simulink model "A320_23b"  (R2024b)
settings: Solver=ode4  StartTime=0.0  StopTime=150  FixedStep=0.001  RelTol=1e-3
InitFcn:
  | % 清空工作区
  | % clear;
  | 
  | % 加载气动数据
  | load('engine_ct_table.mat'); % 或者是你那个存有气动数据的文件名
values from neighbouring files (symbols this model uses):
  a0 = 340.294    [basedata.m]
  alpha_CL_table = [ -3.150;  0.000;  0.139;  0.200;  0.260;  0.290;  0.320;  0.500;  3.150 ]    [basedata.m]
  alpha_Cm_table = [ -3.150; -0.800; -0.400; -0.200; -0.100;  0.000;  0.200;  0.230;  0.260;  0.290;  0.310;  0.400;  0.800;  3.150 ]    [basedata.m]
  alpha_Kde_table = [ -3.141593; -0.698132; -0.349066; -0.174533; -0.087266;  0.000000;  0.087266;  0.174533;  0.349066;  0.698132;  3.141593 ]    [basedata.m]
  b_ref = 35.799979    [basedata.m]
  c_gear = 2 .* damping_ratio .* sqrt(k_gear .* m_eff_gear)    [gear.m]
  c_ref = S_ref / b_ref    (= 3.41891172618)    [basedata.m]
  c_roll = [0.020, 0.018, 0.018]    [gear.m]
  CD0 = 0.01865    [basedata.m]
  CL_D0 = CL_D0_clean    (= 0.175)    [basedata.m]
  CL_table = [  0.000;  0.138;  1.320;  1.480;  1.760;  1.750;  1.600;  1.500;  0.000 ]    [basedata.m]
  Clb = 0.554    [basedata.m]
  Clda = -0.291    [basedata.m]
  CLde = -1.652    [basedata.m]
  Cldr = 0.476    [basedata.m]
  Clp = -2.078    [basedata.m]
  CLq = -57.116    [basedata.m]
  Clr = -2.621    [basedata.m]
  Cm_table = [  0.000; -2.402; -1.861; -0.842; -0.442;  0.000;  1.173;  1.337;  1.489;  1.723;  1.919;  2.276;  2.992;  0.000 ]    [basedata.m]
  Cmde = -11.78    [basedata.m]
  Cmq = -1245.917    [basedata.m]
  Cnb = 1.296    [basedata.m]
  Cnda = -0.007    [basedata.m]
  Cndr = 1.321    [basedata.m]
  Cnp = 0.742    [basedata.m]
  Cnr = -67.303    [basedata.m]
  CSb = -3.252    [basedata.m]
  CSdr = -2.793    [basedata.m]
  CSr = 17.395    [basedata.m]
  CT_ref = 1.3621132    [basedata.m]    (also in generate_engine_ct_table.m)
  CT_table = [      0.000000, 0.000000, 0.000000, 0.000000, 0.000000, 0.000000, 0.000000, 0.000000, 0.000000, 0.000000;      0.091741, 0.057020, 0.052029, 0.028096, -0.017284, -0.037284, -0.057077, -0.205841, -0.315399, -0.488717;      0.142810, 0.072215, 0.053026, 0.030404, -0.009593, -0.026571, -0.041999, -0.151328, -0.266204, -0.439028;      0.189837, 0.082322, 0.055050, 0.032748,  0.017389,  0.003990, -0.0 ...(+1815 chars)    [generate_engine_ct_table.m]
  CYp = 1.833    [basedata.m]
  da_max = 0.436332    [basedata.m]
  da_min = -da_max    (= -0.436332)    [basedata.m]
  de_max = 0.436332    [basedata.m]
  de_min = -0.296706    [basedata.m]
  Delta_CD_flap_tot = 0.1316    [basedata.m]
  Delta_CD_gear = 0.0372    [basedata.m]    (also in gear.m)
  Delta_CD_sp = 0.05775    [basedata.m]
  Delta_CL_flap_tot = 1.867    [basedata.m]
  Delta_CL_sp = -0.466875    [basedata.m]
  Delta_Cm_flap_tot = -0.084    [basedata.m]
  Delta_Cm_gear = 0.0022    [basedata.m]    (also in gear.m)
  Delta_Cm_sp = 0.023    [basedata.m]
  delta_flap_TE_max = 0.698132    [basedata.m]
  delta_flap_TE_tab = [ 0.000000;  0.087266;  0.174533;  0.261799;  0.349066;  0.698132 ]    [basedata.m]
  delta_gear_max = [0.573024, 0.523235, 0.523235]    [gear.m]
  delta_slat_LE_max = 0.471239    [basedata.m]
  delta_slat_LE_tab = [ 0.000000;  0.314159;  0.314334;  0.383972;  0.384147;  0.471239 ]    [basedata.m]
  DH = pi / 180    (= 0.0174532925199)    [basedata.m]
  dr_max = 0.436332    [basedata.m]
  dr_min = -dr_max    (= -0.436332)    [basedata.m]
  g = 9.80665    [basedata.m]
  ground_z = 0.0    (= 0)    [gear.m]
  H_B = H_R - R * cos(a1)    [landing_trajectory.m]
  H_C = H_R - R * cos(a2)    [landing_trajectory.m]
  H_climb_complete = 1000.0    (= 1000)    [landing.m]
  H_entry = 1001    [landing_trajectory.m]
  H_exp = 20    [landing_trajectory.m]
  HD = 180 / pi    (= 57.2957795131)    [basedata.m]
  I = [ Ixx, -Ixy, -Ixz ... (first row only)    [basedata.m]
  K_GE = 1.0    (= 1)    [basedata.m]
  K_gear = F_static_gear ./ (delta_static .^ spring_exp)    [gear.m]
  k_i_eff = 0.07447685    [basedata.m]
  Kde_table = [ -1.000;     0.050;     0.455;     0.853;     1.007;     1.000;     0.839;     0.693;     0.381;    -0.080;   -1.000 ]    [basedata.m]
  lamdaD_flap_TE_tab = [ 0.000;     0.300;     0.630;     0.850;     0.970;     0.939 ]    [basedata.m]
  lamdaD_slat_LE_tab = [ 1.000;     0.330;     0.630;     0.850;     0.970;     0.939 ]    [basedata.m]
  lamdaL_flap_TE_tab = [ 0.000;     0.010;     1.300;     1.300;     1.170;     1.000 ]    [basedata.m]
  lamdaL_slat_LE_tab = [ 1.000;     1.000;     1.000;     1.000;     1.000;     1.000 ]    [basedata.m]
  m = 42500.244    [basedata.m]
  Mach = [0, 0.1, 0.2, 0.3, 0.4, 0.5, 0.6, 0.7, 0.8, 0.9]    [generate_engine_ct_table.m]
  mu_brake = [0.0, 0.55, 0.55]    [gear.m]
  mu_lat = mu_gear    [gear.m]
  N1 = [        0,  20,  25,  30,  35,  40,  45,  50,  55,  60,       65,  70,  75,  80,  85,  90,  95, 100, 105, 110]    [generate_engine_ct_table.m]
  N1_idle = 19.6    [basedata.m]    (also in generate_engine_ct_table.m)
  N1_lim = 101.0    (= 101)    [basedata.m]    (also in generate_engine_ct_table.m)
  phi0 = 0.0    (= 0)    [landing.m]
  psi0 = 0.0    (= 0)    [landing.m]
  r_left_b = r_gear_b(:,2)    [gear.m]
  r_nose_b = r_gear_b(:,1)    [gear.m]
  r_right_b = r_gear_b(:,3)    [gear.m]
  rho0 = 1.225    [basedata.m]
  S_ref = 122.396968    [basedata.m]
  spoiler_max_air = 0.698132    [basedata.m]
  spring_exp = [2.05, 1.05, 1.05]    [gear.m]
  T_static = 120635.770206    [basedata.m]    (also in generate_engine_ct_table.m)
  theta0 = alpha_trim    [landing.m]
  V_app = 1.4 * Vs    [landing_trajectory.m]
  V_cruise = 234.072222    [basedata.m]
  v_eps = 0.20    (= 0.2)    [gear.m]
  V_flare = 1.4 * V_stall_full    (= 82.8255554)    [basedata.m]    (also in landing.m = 1.4 * V_stall_full)
  V_lat_ref = 0.20    (= 0.2)    [gear.m]
  V_min = 3    [landing.m]
  V_shallow = 1.2 * Vs    [landing_trajectory.m]
  wheel_radius = [0.381000, 0.584210, 0.584210]    [gear.m]
  WOW_on = 0.005    [gear.m]
  X_landing_start = -11500    [landing.m]
  Xg0 = -11500.0    (= -11500)    [landing.m]
  Yg0 = 100.0    (= 100)    [landing.m]
  Zg0 = -10000    [gear.m]    (also in landing.m = -1000)
undefined symbols (not defined in the file or in its folder): I_xz, I_yz, Ix_Iy, Iy_Iz, Iz_Ix
libraries: simulink x51, matrix_library x19
(part 1 of 3)
settings Model: SimulationMode=accelerator  Creator=34355  LastModifiedBy=34355

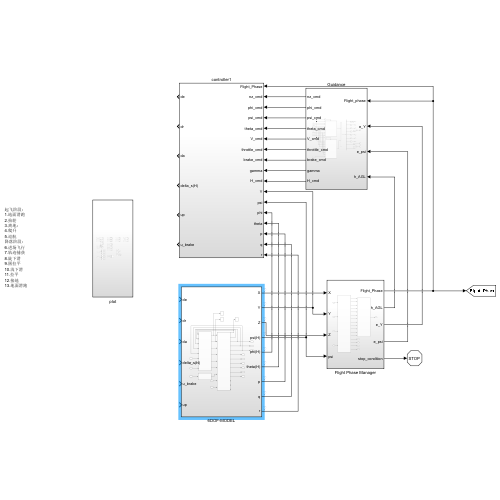
[thumbnail: Simulink's stored preview of the top-level diagram]
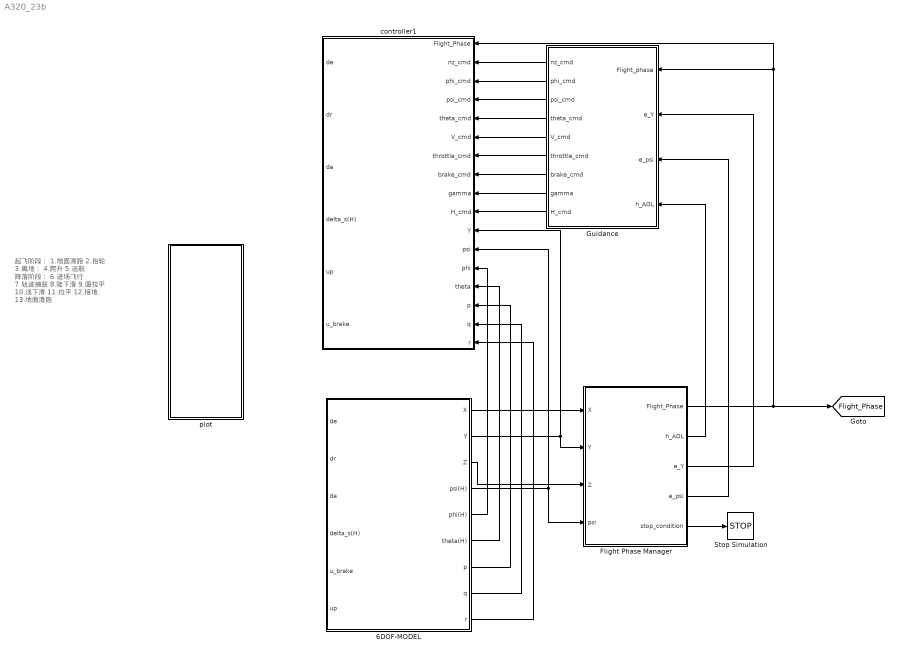
== system A320_23b ==
  note: 起飞阶段：
      | 1.地面滑跑
      | 2.抬轮
      | 3.离地：
      | 4.爬升
      | 5.巡航
      | 降落阶段：
      | 6.进场飞行
      | 7.轨迹捕获
      | 8.陡下滑
      | 9.圆拉平
      | 10.浅下滑
      | 11.拉平
      | 12.接地
      | 13.地面滑跑
  6DOF-MODEL : Subsystem
  Flight Phase Manager : Subsystem
  Guidance : Subsystem
  Stop Simulation : Stop
  controller1 : Subsystem
  plot : Subsystem
  tag scope: Flight_Phase=global
  wires:
  Flight Phase Manager/1(Flight_Phase) -> [Flight_Phase], Guidance/1(Flight_phase), controller1/1(Flight_Phase)
  Flight Phase Manager/3(e_Y) -> Guidance/2(e_Y)
  Flight Phase Manager/4(e_psi) -> Guidance/3(e_psi)
  Flight Phase Manager/2(h_AGL) -> Guidance/4(h_AGL)
  Guidance/1(nz_cmd) -> controller1/2(nz_cmd)
  Guidance/2(phi_cmd) -> controller1/3(phi_cmd)
  Guidance/4(theta_cmd) -> controller1/5(theta_cmd)
  Guidance/5(V_cmd) -> controller1/6(V_cmd)
  Guidance/6(throttle_cmd) -> controller1/7(throttle_cmd)
  Guidance/7(brake_cmd) -> controller1/8(brake_cmd)
  Guidance/8(gamma) -> controller1/9(gamma)
  Guidance/9(H_cmd) -> controller1/10(H_cmd)
  Flight Phase Manager/5(stop_condition) -> Stop Simulation/1
  Guidance/3(psi_cmd) -> controller1/4(psi_cmd)
  6DOF-MODEL/1(X) -> Flight Phase Manager/1(X)
  6DOF-MODEL/2(Y) -> controller1/11(Y), Flight Phase Manager/2(Y)
  6DOF-MODEL/3(Z) -> Flight Phase Manager/3(Z)
  6DOF-MODEL/4(psi(H)) -> Flight Phase Manager/4(psi), controller1/12(psi)
  6DOF-MODEL/5(phi(H)) -> controller1/13(phi)
  6DOF-MODEL/6(theta(H)) -> controller1/14(theta)
  6DOF-MODEL/7(p) -> controller1/15(p)
  6DOF-MODEL/8(q) -> controller1/16(q)
  6DOF-MODEL/9(r) -> controller1/17(r)

== system A320_23b/6DOF-MODEL ==
  de : Inport
  dr : Inport  Port=2
  da : Inport  Port=3
  delta_s(H) : Inport  Port=4
  u_brake : Inport  Port=5
  up : Inport  Port=6
  AERO-PARAMETER : Subsystem
  Scope : Scope
  Scope5 : Scope
  Scope6 : Scope
  动力学 : Subsystem
  发动机 : Subsystem
  X : Outport
  Y : Outport  Port=2
  Z : Outport  Port=3
  psi(H) : Outport  Port=4
  phi(H) : Outport  Port=5
  theta(H) : Outport  Port=6
  p : Outport  Port=7
  q : Outport  Port=8
  r : Outport  Port=9
  wires:
  动力学/1(alpha(D)) -> Scope/1, AERO-PARAMETER/1(alpha(D))
  发动机/1(T) -> 动力学/7(thrust)
  u_brake/1 -> 动力学/9(u_brake)
  AERO-PARAMETER/1(D) -> Scope6/1, 动力学/1(D)
  AERO-PARAMETER/2(L) -> Scope5/1, 动力学/2(L)
  AERO-PARAMETER/3(S) -> 动力学/3(S)
  AERO-PARAMETER/4(MX) -> 动力学/4(MX)
  AERO-PARAMETER/5(MY) -> 动力学/5(MY)
  AERO-PARAMETER/6(MZ) -> 动力学/6(MZ)
  delta_s(H)/1 -> 动力学/8(delta_s(H))
  动力学/2(beta(D)) -> AERO-PARAMETER/2(beta(D))
  动力学/3(p) -> p/1, AERO-PARAMETER/3(p(H))
  动力学/4(q) -> q/1, AERO-PARAMETER/4(q(H))
  动力学/5(r) -> r/1, AERO-PARAMETER/5(r(H))
  de/1 -> AERO-PARAMETER/6(de(D))
  dr/1 -> AERO-PARAMETER/7(dr(D))
  da/1 -> AERO-PARAMETER/8(da)
  动力学/7(Y) -> Y/1
  动力学/8(Z) -> Z/1
  动力学/11(psi(H)) -> psi(H)/1
  动力学/10(theta(H)) -> theta(H)/1
  动力学/6(X) -> X/1
  动力学/9(phi(H)) -> phi(H)/1
  up/1 -> 发动机/1(up)

== system A320_23b/Flight Phase Manager ==
  X : Inport
  Y : Inport  Port=2
  Z : Inport  Port=3
  psi : Inport  Port=4
  Data Pre-processing : Subsystem
  Phase Logic : Stateflow chart  TreatAsAtomicUnit=on
  Flight_Phase : Outport
  h_AGL : Outport  Port=2
  e_Y : Outport  Port=3
  e_psi : Outport  Port=4
  stop_condition : Outport  Port=5
  wires:
  X/1 -> Data Pre-processing/1(X)
  Y/1 -> Data Pre-processing/2(Y)
  Z/1 -> Data Pre-processing/3(Z)
  psi/1 -> Data Pre-processing/4(psi)
  Phase Logic/1(Flight_Phase) -> Flight_Phase/1
  Data Pre-processing/1(reach_VR) -> Phase Logic/1(reach_VR)
  Data Pre-processing/2(airborne) -> Phase Logic/2(airborne)
  Data Pre-processing/3(safe_climb) -> Phase Logic/3(safe_climb)
  Data Pre-processing/4(in_cruise) -> Phase Logic/4(in_cruise)
  Data Pre-processing/5(task_mode) -> Phase Logic/5(Task_Mode)
  Data Pre-processing/6(Trajectory_capture) -> Phase Logic/6(Trajectory_capture)
  Data Pre-processing/7(in_steep) -> Phase Logic/7(in_steep)
  Data Pre-processing/8(In_round) -> Phase Logic/8(in_round)
  Data Pre-processing/9(Slight decline) -> Phase Logic/9(Slight_decline)
  Data Pre-processing/10(in_flare) -> Phase Logic/10(in_Flare)
  Data Pre-processing/11(touch_ground) -> Phase Logic/11(touch_ground)
  Data Pre-processing/12(in_ground) -> Phase Logic/12(in_ground)
  Data Pre-processing/13(h_ALG) -> h_AGL/1
  Data Pre-processing/15(e_Y) -> e_Y/1
  Data Pre-processing/14(e_psi) -> e_psi/1
  Data Pre-processing/16(stop_condition) -> stop_condition/1

== system A320_23b/Guidance ==
  Flight_phase : Inport
  e_Y : Inport  Port=2
  e_psi : Inport  Port=3
  h_AGL : Inport  Port=4
  Bus Selector : BusSelector  OutputSignals=nz_cmd,phi_cmd,psi_cmd,theta_cmd,V_cmd,throttle_cmd,brake_cmd,H_cmd,gamma
  Compare To Constant : simulink/Logic and Bit Operations/Compare To Constant  relop=<=  const=5  OutDataTypeStr=boolean
  Compare To Constant1 : simulink/Logic and Bit Operations/Compare To Constant  relop=>  const=5  OutDataTypeStr=boolean
  Gain : Gain  Gain=HD
  Gain1 : Gain  Gain=HD
  Merge : Merge
  Rate Limiter : RateLimiter  RisingSlewLimit=1*DH  FallingSlewLimit=-1*DH  SampleTimeMode=inherited
  Rate Limiter1 : RateLimiter  RisingSlewLimit=10*DH  FallingSlewLimit=-10*DH  SampleTimeMode=inherited
  Rate Limiter2 : RateLimiter  RisingSlewLimit=10*DH  FallingSlewLimit=-10*DH  SampleTimeMode=inherited
  Rate Limiter3 : RateLimiter  RisingSlewLimit=0.8  FallingSlewLimit=-0.8  SampleTimeMode=inherited
  Saturation : Saturate  UpperLimit=2  LowerLimit=-2
  Saturation2 : Saturate  UpperLimit=1  LowerLimit=0
  Saturation3 : Saturate  UpperLimit=1  LowerLimit=0
  Saturation4 : Saturate  UpperLimit=250  LowerLimit=0
  Scope : Scope
  Scope8 : Scope
  Scope9 : Scope
  起飞阶段 : Subsystem
  降落阶段 : Subsystem
  nz_cmd : Outport
  phi_cmd : Outport  Port=2
  psi_cmd : Outport  Port=3
  theta_cmd : Outport  Port=4
  V_cmd : Outport  Port=5
  throttle_cmd : Outport  Port=6
  brake_cmd : Outport  Port=7
  gamma : Outport  Port=8
  H_cmd : Outport  Port=9
  wires:
  Bus Selector/5 -> Saturation4/1  "<V_cmd>"
  Bus Selector/4 -> Rate Limiter/1  "<theta_cmd>"
  Saturation4/1 -> V_cmd/1
  Bus Selector/7 -> Saturation3/1  "<brake_cmd>"
  Rate Limiter2/1 -> psi_cmd/1
  Saturation/1 -> Rate Limiter3/1
  Saturation3/1 -> brake_cmd/1
  Saturation2/1 -> throttle_cmd/1
  Merge/1 -> Bus Selector/1
  [vzg] -> 起飞阶段/8(vzg), 降落阶段/6(vzg)
  Rate Limiter/1 -> theta_cmd/1, Gain1/1
  Bus Selector/2 -> Rate Limiter1/1  "<phi_cmd>"
  Bus Selector/8 -> H_cmd/1, Scope9/1  "<H_cmd>"
  [theta_eular] -> 降落阶段/8(theta_eular), 起飞阶段/10(theta_eular)
  降落阶段/1(Cmd_Bus) -> Merge/2
  Bus Selector/1 -> Saturation/1  "<nz_cmd>"
  h_AGL/1 -> 起飞阶段/7(h_ALG), 降落阶段/2(h_AGL)
  [vxg] -> 降落阶段/9(Vg)
  [phi_eular] -> 起飞阶段/9(phi_eular), 降落阶段/7(phi_eular)
  起飞阶段/1(Cmd_Bus) -> Merge/1
  Flight_phase/1 -> Compare To Constant/1, 起飞阶段/1(Flight_phase), 降落阶段/1(Flight_phase), Compare To Constant1/1
  Compare To Constant/1 -> 起飞阶段/Enable
  [r] -> 起飞阶段/4(r)
  [Vwind_ground] -> 起飞阶段/5(Vwind_ground), 降落阶段/3(Vwind_ground)
  e_psi/1 -> 起飞阶段/3(e_psi)
  Gain/1 -> Scope8/1
  e_Y/1 -> 起飞阶段/2(e_Y)
  Bus Selector/9 -> gamma/1, Gain/1  "<gamma>"
  Compare To Constant1/1 -> 降落阶段/Enable
  [Va_safe] -> 起飞阶段/6(Va_safe), 降落阶段/4(Va_safe)
  Rate Limiter3/1 -> nz_cmd/1
  Bus Selector/6 -> Saturation2/1  "<throttle_cmd>"
  Rate Limiter1/1 -> phi_cmd/1
  [X_positon] -> 降落阶段/5(x_pos)
  Bus Selector/3 -> Rate Limiter2/1  "<psi_cmd>"
  Gain1/1 -> Scope/1

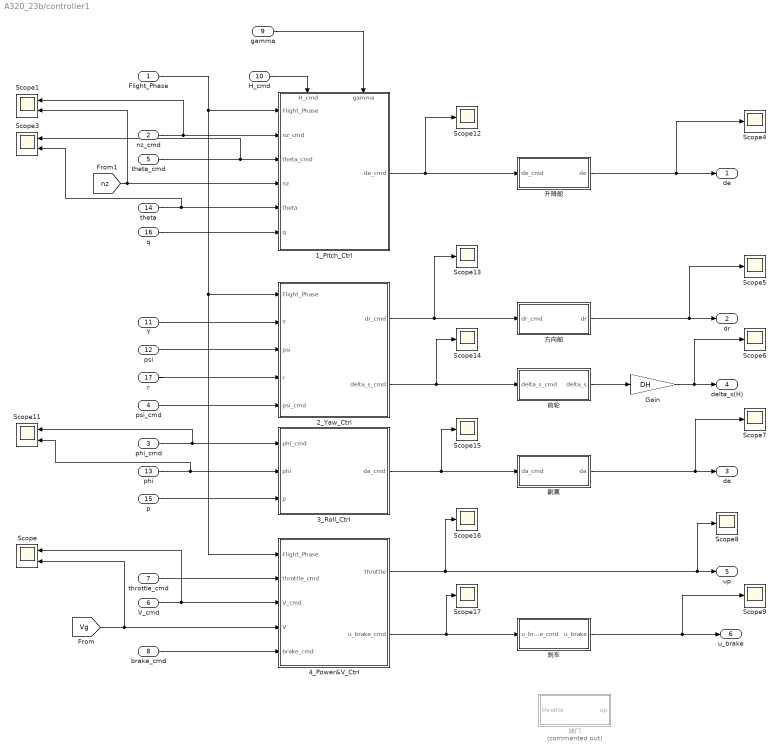
== system A320_23b/controller1 ==
  Flight_Phase : Inport
  nz_cmd : Inport  Port=2
  phi_cmd : Inport  Port=3
  psi_cmd : Inport  Port=4
  theta_cmd : Inport  Port=5
  V_cmd : Inport  Port=6
  throttle_cmd : Inport  Port=7
  brake_cmd : Inport  Port=8
  gamma : Inport  Port=9
  H_cmd : Inport  Port=10
  Y : Inport  Port=11
  psi : Inport  Port=12
  phi : Inport  Port=13
  theta : Inport  Port=14
  p : Inport  Port=15
  q : Inport  Port=16
  r : Inport  Port=17
  1_Pitch_Ctrl : Subsystem
      settings: PortSchema="{\"entries\":[{\"content\":{\"sides\":[{\"content\":{\"connectorIds\":[\"In1\",\"In2\",\"In3\",\"In4\",\"In5\",\"In6\"]},\"type\":\"ConnectorPlacement.EquallySpacedRectSide\",\"uuid\":\"27d13232-9f89-4ac1-9c77-5758657de7c7\"},{\"content\":{\"connectorIds\":[\"Out1\"],\"side\":\"RIGHT\"},\"type\":\"ConnectorPlacement.EquallySpacedRectSide\",\"uuid\":\"ae62ad8c-a405-4422-b5ec-9ac723f70591\"},{\"content\":{\"connectorIds\":[\"In7\",\"In8\"],\"side\":\"TOP\"},\"type\":\"ConnectorPlacement.EquallySpacedRectSide\",\"uuid\":\"4cebe0f4-d768-4fb6-931c-2fd4183255b7\"}]},\"type\":\"ConnectorPlacement.EquallySpacedConnector\",\"uuid\":\"2c44e0df-7f94-4dab-9232-216c905b911f\"}],\"packageUris\":[\"http://schema.mathworks.com/mf0/Connector/R2020b\"],\"version\":\"1.0\"}"
  2_Yaw_Ctrl : Subsystem
  3_Roll_Ctrl : Subsystem
  4_Power&V_Ctrl : Subsystem
  Gain : Gain  Gain=DH
  Scope{,1,3,11} (4 alike) : Scope  NumInputPorts=2
  Scope{4..9,12..17} (12 alike) : Scope
  刹车 : Subsystem
  前轮 : Subsystem
  副翼 : Subsystem
  升降舵 : Subsystem
  方向舵 : Subsystem
  油门 : Subsystem  Commented=on
  de : Outport
  dr : Outport  Port=2
  da : Outport  Port=3
  delta_s(H) : Outport  Port=4
  up : Outport  Port=5
  u_brake : Outport  Port=6
  wires:
  phi_cmd/1 -> Scope11/1, 3_Roll_Ctrl/1(phi_cmd)
  phi/1 -> Scope11/2, 3_Roll_Ctrl/2(phi)
  p/1 -> 3_Roll_Ctrl/3(p)
  brake_cmd/1 -> 4_Power&V_Ctrl/5(brake_cmd)
  4_Power&V_Ctrl/1(throttle) -> Scope8/1, up/1, Scope16/1
  Flight_Phase/1 -> 1_Pitch_Ctrl/1(Flight_Phase), 4_Power&V_Ctrl/1(Flight_Phase), 2_Yaw_Ctrl/1(Flight_Phase)
  nz_cmd/1 -> 1_Pitch_Ctrl/2(nz_cmd), Scope1/1
  [nz] -> 1_Pitch_Ctrl/4(nz), Scope1/2
  q/1 -> 1_Pitch_Ctrl/6(q)
  V_cmd/1 -> Scope/1, 4_Power&V_Ctrl/3(V_cmd)
  [Vg] -> Scope/2, 4_Power&V_Ctrl/4(V)
  Gain/1 -> Scope6/1, delta_s(H)/1
  theta_cmd/1 -> 1_Pitch_Ctrl/3(theta_cmd), Scope3/1
  1_Pitch_Ctrl/1(de_cmd) -> 升降舵/1(de_cmd), Scope12/1
  2_Yaw_Ctrl/1(dr_cmd) -> Scope13/1, 方向舵/1(dr_cmd)
  2_Yaw_Ctrl/2(delta_s_cmd) -> Scope14/1, 前轮/1(delta_s_cmd)
  3_Roll_Ctrl/1(da_cmd) -> Scope15/1, 副翼/1(da_cmd)
  4_Power&V_Ctrl/2(u_brake_cmd) -> Scope17/1, 刹车/1(u_brake_cmd)
  theta/1 -> 1_Pitch_Ctrl/5(theta), Scope3/2
  throttle_cmd/1 -> 4_Power&V_Ctrl/2(throttle_cmd)
  Y/1 -> 2_Yaw_Ctrl/2(Y)
  psi/1 -> 2_Yaw_Ctrl/3(psi)
  r/1 -> 2_Yaw_Ctrl/4(r)
  升降舵/1(de) -> Scope4/1, de/1
  方向舵/1(dr) -> Scope5/1, dr/1
  前轮/1(delta_s) -> Gain/1
  副翼/1(da) -> Scope7/1, da/1
  刹车/1(u_brake) -> Scope9/1, u_brake/1
  H_cmd/1 -> 1_Pitch_Ctrl/7(H_cmd)
  gamma/1 -> 1_Pitch_Ctrl/8(gamma)
  psi_cmd/1 -> 2_Yaw_Ctrl/5(psi_cmd)

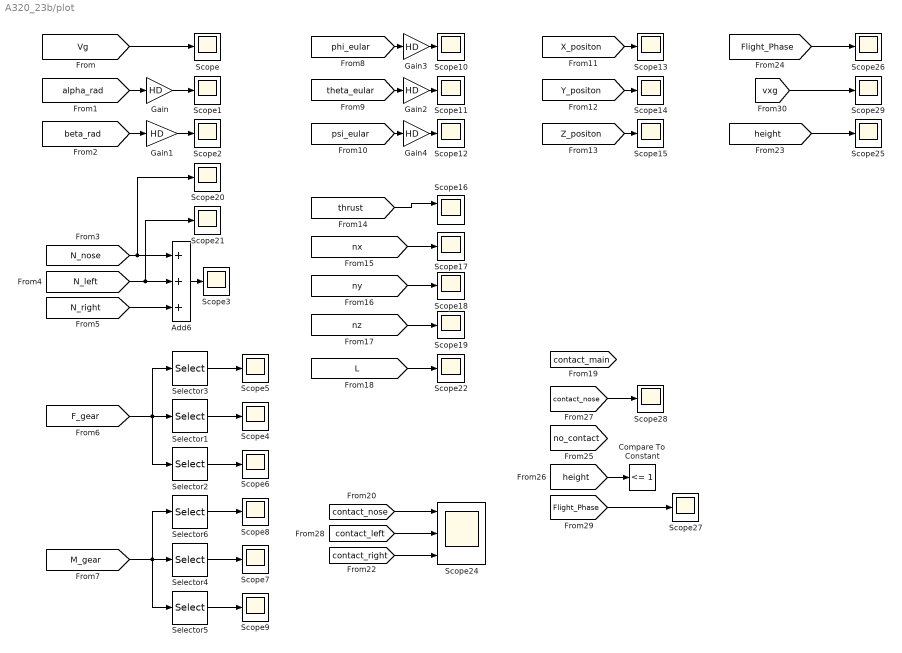
== system A320_23b/plot ==
  Add6 : Sum  Inputs=+++
  Compare To Constant : simulink/Logic and Bit Operations/Compare To Constant  relop=<=  const=1  OutDataTypeStr=boolean
  Gain{,1..4} (5 alike) : Gain  Gain=HD
  Scope{,1..15,17..22,25..29} (27 alike) : Scope
  Scope16 : Scope  NumInputPorts=2
  Scope24 : Scope  NumInputPorts=3
  Selector1 : Selector  InputPortWidth=3  IndexOptions=Index vector (dialog)  Indices=2  OutputSizes=1
  Selector2 : Selector  InputPortWidth=3  IndexOptions=Index vector (dialog)  Indices=3  OutputSizes=1
  Selector3 : Selector  InputPortWidth=3  IndexOptions=Index vector (dialog)  Indices=1  OutputSizes=1
  Selector4 : Selector  InputPortWidth=3  IndexOptions=Index vector (dialog)  Indices=2  OutputSizes=1
  Selector5 : Selector  InputPortWidth=3  IndexOptions=Index vector (dialog)  Indices=3  OutputSizes=1
  Selector6 : Selector  InputPortWidth=3  IndexOptions=Index vector (dialog)  Indices=1  OutputSizes=1
  wires:
  [N_nose] -> Add6/1, Scope20/1
  [N_left] -> Scope21/1, Add6/2
  [N_right] -> Add6/3
  [Vg] -> Scope/1
  [alpha_rad] -> Gain/1
  [beta_rad] -> Gain1/1
  Add6/1 -> Scope3/1
  Selector3/1 -> Scope5/1
  Selector2/1 -> Scope6/1
  Selector1/1 -> Scope4/1
  [F_gear] -> Selector2/1, Selector1/1, Selector3/1
  Selector6/1 -> Scope8/1
  Selector4/1 -> Scope7/1
  [M_gear] -> Selector6/1, Selector4/1, Selector5/1
  Selector5/1 -> Scope9/1
  [psi_eular] -> Gain4/1
  [theta_eular] -> Gain2/1
  [phi_eular] -> Gain3/1
  Gain1/1 -> Scope2/1
  Gain/1 -> Scope1/1
  Gain2/1 -> Scope11/1
  [Y_positon] -> Scope14/1
  [X_positon] -> Scope13/1
  [Z_positon] -> Scope15/1
  Gain3/1 -> Scope10/1
  Gain4/1 -> Scope12/1
  [thrust] -> Scope16/1
  [nx] -> Scope17/1
  [ny] -> Scope18/1
  [nz] -> Scope19/1
  [L] -> Scope22/1
  [height] -> Scope25/1
  [height] -> Compare To Constant/1
  [contact_left] -> Scope24/2
  [contact_right] -> Scope24/3
  [Flight_Phase] -> Scope26/1
  [contact_nose] -> Scope28/1
  [contact_nose] -> Scope24/1
  [Flight_Phase] -> Scope27/1
  [vxg] -> Scope29/1

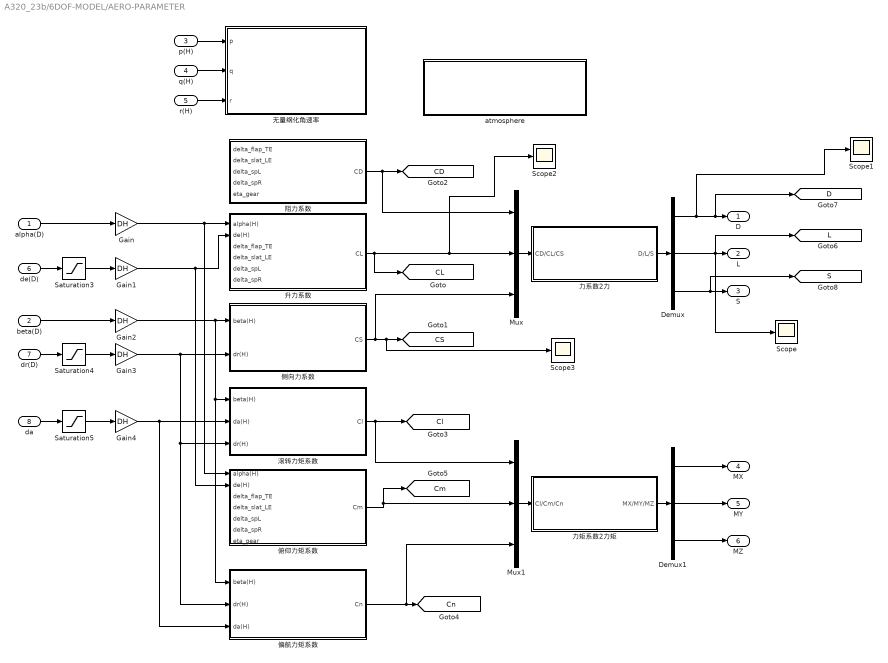
== system A320_23b/6DOF-MODEL/AERO-PARAMETER ==
  alpha(D) : Inport
  beta(D) : Inport  Port=2
  p(H) : Inport  Port=3
  q(H) : Inport  Port=4
  r(H) : Inport  Port=5
  de(D) : Inport  Port=6
  dr(D) : Inport  Port=7
  da : Inport  Port=8
  Demux : Demux  Outputs=3
  Demux1 : Demux  Outputs=3
  Gain{,1..4} (5 alike) : Gain  Gain=DH
  Mux : Mux  Inputs=3
  Mux1 : Mux  Inputs=3
  Saturation3 : Saturate  UpperLimit=de_max  LowerLimit=de_min
  Saturation4 : Saturate  UpperLimit=dr_max  LowerLimit=dr_min
  Saturation5 : Saturate  UpperLimit=da_max  LowerLimit=da_min
  Scope{,1..3} (4 alike) : Scope
  atmosphere : Subsystem
  侧向力系数 : Subsystem
  俯仰力矩系数 : Subsystem
  偏航力矩系数 : Subsystem
  力矩系数2力矩 : Subsystem
  力系数2力 : Subsystem
  升力系数 : Subsystem
  无量纲化角速率 : Subsystem
  滚转力矩系数 : Subsystem
  阻力系数 : Subsystem
  D : Outport
  L : Outport  Port=2
  S : Outport  Port=3
  MX : Outport  Port=4
  MY : Outport  Port=5
  MZ : Outport  Port=6
  tag scope: CD=global, CL=global, CS=global, Cl=global, Cm=global, Cn=global, D=global, L=global, S=global
  wires:
  升力系数/1(CL) -> [CL], Scope2/1, Mux/2
  侧向力系数/1(CS) -> Mux/3, Scope3/1, [CS]
  da/1 -> Saturation5/1
  Saturation5/1 -> Gain4/1
  Saturation4/1 -> Gain3/1
  dr(D)/1 -> Saturation4/1
  de(D)/1 -> Saturation3/1
  Saturation3/1 -> Gain1/1
  beta(D)/1 -> Gain2/1
  alpha(D)/1 -> Gain/1
  Gain/1 -> 俯仰力矩系数/1(alpha(H)), 升力系数/1(alpha(H))
  Gain1/1 -> 俯仰力矩系数/2(de(H)), 升力系数/2(de(H))
  Gain2/1 -> 侧向力系数/1(beta(H)), 偏航力矩系数/1(beta(H)), 滚转力矩系数/1(beta(H))
  Gain3/1 -> 侧向力系数/2(dr(H)), 偏航力矩系数/2(dr(H)), 滚转力矩系数/3(dr(H))
  Gain4/1 -> 偏航力矩系数/3(da(H)), 滚转力矩系数/2(da(H))
  p(H)/1 -> 无量纲化角速率/1(p)
  q(H)/1 -> 无量纲化角速率/2(q)
  r(H)/1 -> 无量纲化角速率/3(r)
  阻力系数/1(CD) -> Mux/1, [CD]
  滚转力矩系数/1(Cl) -> [Cl], Mux1/1
  俯仰力矩系数/1(Cm) -> Mux1/2, [Cm]
  偏航力矩系数/1(Cn) -> Mux1/3, [Cn]
  Mux/1 -> 力系数2力/1(CD/CL/CS)
  Mux1/1 -> 力矩系数2力矩/1(Cl/Cm/Cn)
  Demux/2 -> Scope/1, [L], L/1
  力系数2力/1(D/L/S) -> Demux/1
  Demux/1 -> Scope1/1, [D], D/1
  Demux/3 -> [S], S/1
  力矩系数2力矩/1(MX/MY/MZ) -> Demux1/1
  Demux1/1 -> MX/1
  Demux1/2 -> MY/1
  Demux1/3 -> MZ/1

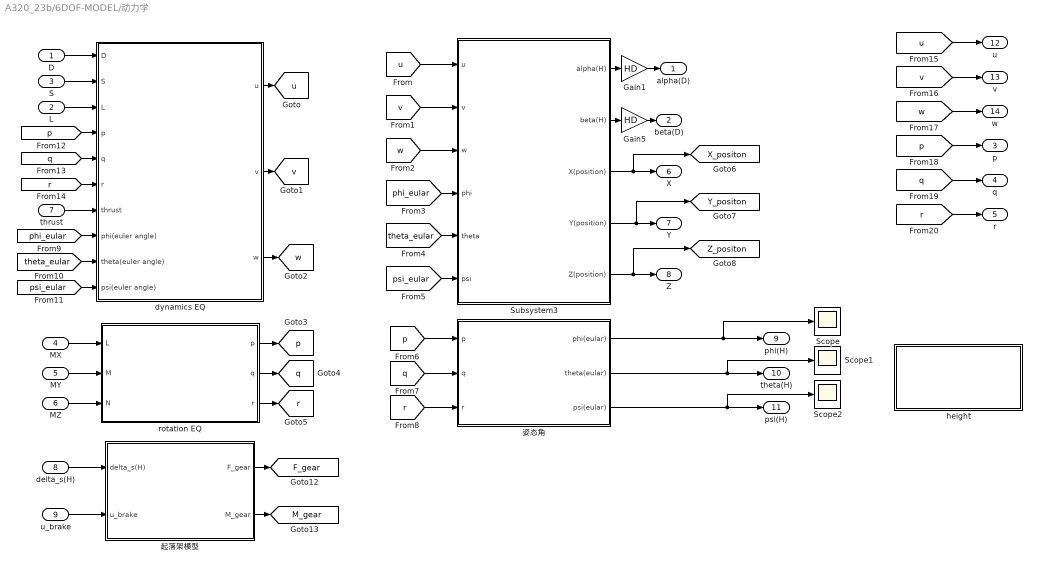
== system A320_23b/6DOF-MODEL/动力学 ==
  D : Inport
  L : Inport  Port=2
  S : Inport  Port=3
  MX : Inport  Port=4
  MY : Inport  Port=5
  MZ : Inport  Port=6
  thrust : Inport  Port=7
  delta_s(H) : Inport  Port=8
  u_brake : Inport  Port=9
  Gain1 : Gain  Gain=HD
  Gain5 : Gain  Gain=HD
  Scope : Scope
  Scope1 : Scope
  Scope2 : Scope
  Subsystem3 : Subsystem
  dynamics EQ : Subsystem
  height : Subsystem
  rotation EQ : Subsystem
  姿态角 : Subsystem
  起落架模型 : Subsystem
  alpha(D) : Outport
  beta(D) : Outport  Port=2
  p : Outport  Port=3
  q : Outport  Port=4
  r : Outport  Port=5
  X : Outport  Port=6
  Y : Outport  Port=7
  Z : Outport  Port=8
  phi(H) : Outport  Port=9
  theta(H) : Outport  Port=10
  psi(H) : Outport  Port=11
  u : Outport  Port=12
  v : Outport  Port=13
  w : Outport  Port=14
  tag scope: F_gear=global, M_gear=global, X_positon=global, Y_positon=global, Z_positon=global, p=global, q=global, r=global, u=global, v=global, w=global
  wires:
  姿态角/1(phi(eular)) -> Scope/1, phi(H)/1
  姿态角/2(theta(eular)) -> theta(H)/1, Scope1/1
  姿态角/3(psi(eular)) -> psi(H)/1, Scope2/1
  Gain5/1 -> beta(D)/1
  Gain1/1 -> alpha(D)/1
  [u] -> u/1
  [v] -> v/1
  [w] -> w/1
  [p] -> p/1
  [q] -> q/1
  [r] -> r/1
  起落架模型/1(F_gear) -> [F_gear]
  起落架模型/2(M_gear) -> [M_gear]
  MX/1 -> rotation EQ/1(L)
  MY/1 -> rotation EQ/2(M)
  MZ/1 -> rotation EQ/3(N)
  D/1 -> dynamics EQ/1(D)
  S/1 -> dynamics EQ/2(S)
  L/1 -> dynamics EQ/3(L)
  [p] -> dynamics EQ/4(p)
  [q] -> dynamics EQ/5(q)
  [r] -> dynamics EQ/6(r)
  thrust/1 -> dynamics EQ/7(thrust)
  [phi_eular] -> dynamics EQ/8(phi(euler angle))
  [theta_eular] -> dynamics EQ/9(theta(euler angle))
  [psi_eular] -> dynamics EQ/10(psi(euler angle))
  dynamics EQ/1(u) -> [u]
  dynamics EQ/2(v) -> [v]
  dynamics EQ/3(w) -> [w]
  [u] -> Subsystem3/1(u)
  [v] -> Subsystem3/2(v)
  [w] -> Subsystem3/3(w)
  [phi_eular] -> Subsystem3/4(phi)
  [theta_eular] -> Subsystem3/5(theta)
  [psi_eular] -> Subsystem3/6(psi)
  Subsystem3/1(alpha(H)) -> Gain1/1
  Subsystem3/2(beta(H)) -> Gain5/1
  Subsystem3/3(X(position)) -> [X_positon], X/1
  Subsystem3/4(Y(position)) -> [Y_positon], Y/1
  Subsystem3/5(Z(position)) -> [Z_positon], Z/1
  delta_s(H)/1 -> 起落架模型/1(delta_s(H))
  u_brake/1 -> 起落架模型/2(u_brake)
  rotation EQ/1(p) -> [p]
  rotation EQ/2(q) -> [q]
  rotation EQ/3(r) -> [r]
  [p] -> 姿态角/1(p)
  [q] -> 姿态角/2(q)
  [r] -> 姿态角/3(r)

== system A320_23b/6DOF-MODEL/发动机 ==
  up : Inport
  2-D Lookup Table : Lookup_n-D  BreakpointsForDimension1=N1  BreakpointsForDimension2=Mach  Table=CT_table  InternalRulePriority=Speed  RndMeth=Simplest
      settings: InputPortMap=u0,u1
  Add : Sum
  Add1 : Sum  Inputs=+-
  Constant1 : Constant  Value=T_static
  Constant2 : Constant  Value=CT_ref
  Constant5 : Constant  Value=0
  Constant6 : Constant  Value=N1_idle
  Constant7 : Constant  Value=N1_lim
  Divide : Product  Inputs=**/
  Gain1 : Gain  Gain=2
  Multiport Switch : MultiPortSwitch  DataPortOrder=Zero-based contiguous  zeroidx=on  SaturateOnIntegerOverflow=off  InputSameDT=off
  Product1 : Product
  Scope{,1..4} (5 alike) : Scope
  状态012 : Constant  Value=2
  T : Outport
  tag scope: thrust=global
  wires:
  Constant6/1 -> Add1/2, Add/1, Multiport Switch/3
  Constant1/1 -> Divide/1
  Add1/1 -> Product1/2
  Constant2/1 -> Divide/3
  Divide/1 -> Gain1/1
  Gain1/1 -> Scope1/1, [thrust], T/1
  Add/1 -> Multiport Switch/4
  2-D Lookup Table/1 -> Divide/2, Scope2/1
  Constant5/1 -> Multiport Switch/2
  up/1 -> Scope/1, Product1/1
  [mach] -> Scope4/1, 2-D Lookup Table/2
  Multiport Switch/1 -> Scope3/1, 2-D Lookup Table/1
  Constant7/1 -> Add1/1
  Product1/1 -> Add/2
  状态012/1 -> Multiport Switch/1

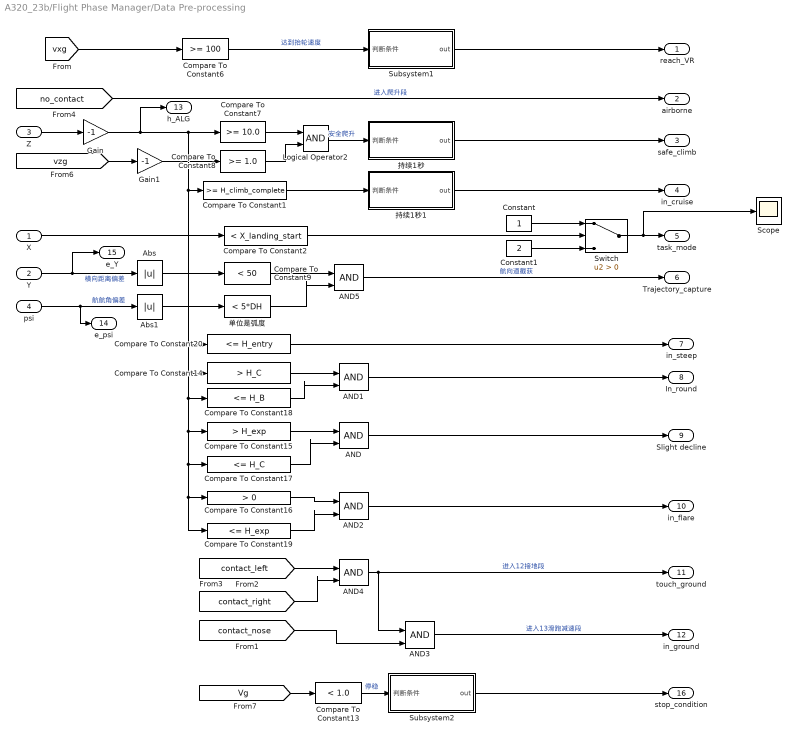
== system A320_23b/Flight Phase Manager/Data Pre-processing ==
  X : Inport
  Y : Inport  Port=2
  Z : Inport  Port=3
  psi : Inport  Port=4
  AND{,1..5} (6 alike) : Logic  IconShape=distinctive  AllPortsSameDT=off  OutDataTypeStr=boolean
  Abs : Abs  SaturateOnIntegerOverflow=off
  Abs1 : Abs  SaturateOnIntegerOverflow=off
  Compare To Constant1 : simulink/Logic and Bit Operations/Compare To Constant  relop=>=  const=H_climb_complete  OutDataTypeStr=boolean
  Compare To Constant13 : simulink/Logic and Bit Operations/Compare To Constant  relop=<  const=1.0  OutDataTypeStr=boolean
  Compare To Constant14 : simulink/Logic and Bit Operations/Compare To Constant  relop=>  const=H_C  OutDataTypeStr=boolean
  Compare To Constant15 : simulink/Logic and Bit Operations/Compare To Constant  relop=>  const=H_exp  OutDataTypeStr=boolean
  Compare To Constant16 : simulink/Logic and Bit Operations/Compare To Constant  relop=>  const=0  OutDataTypeStr=boolean
  Compare To Constant17 : simulink/Logic and Bit Operations/Compare To Constant  relop=<=  const=H_C  OutDataTypeStr=boolean
  Compare To Constant18 : simulink/Logic and Bit Operations/Compare To Constant  relop=<=  const=H_B  OutDataTypeStr=boolean
  Compare To Constant19 : simulink/Logic and Bit Operations/Compare To Constant  relop=<=  const=H_exp  OutDataTypeStr=boolean
  Compare To Constant2 : simulink/Logic and Bit Operations/Compare To Constant  relop=<  const=X_landing_start  OutDataTypeStr=boolean
  Compare To Constant20 : simulink/Logic and Bit Operations/Compare To Constant  relop=<=  const=H_entry  OutDataTypeStr=boolean
  Compare To Constant6 : simulink/Logic and Bit Operations/Compare To Constant  relop=>=  const=100  OutDataTypeStr=boolean
  Compare To Constant7 : simulink/Logic and Bit Operations/Compare To Constant  relop=>=  const=10.0  OutDataTypeStr=boolean
  Compare To Constant8 : simulink/Logic and Bit Operations/Compare To Constant  relop=>=  const=1.0  OutDataTypeStr=boolean
  Compare To Constant9 : simulink/Logic and Bit Operations/Compare To Constant  relop=<  const=50  OutDataTypeStr=boolean
  Constant : Constant
  Constant1 : Constant  Value=2
  Gain : Gain  Gain=-1
  Gain1 : Gain  Gain=-1
  Logical Operator2 : Logic  AllPortsSameDT=off  OutDataTypeStr=boolean
  Scope : Scope
  Subsystem1 : Subsystem
  Subsystem2 : Subsystem
  Switch : Switch  Criteria=u2 > Threshold  SaturateOnIntegerOverflow=off  InputSameDT=off
  单位是弧度 : simulink/Logic and Bit Operations/Compare To Constant  relop=<  const=5*DH  OutDataTypeStr=boolean
  持续1秒 : Subsystem
  持续1秒1 : Subsystem
  reach_VR : Outport
  airborne : Outport  Port=2
  safe_climb : Outport  Port=3
  in_cruise : Outport  Port=4
  task_mode : Outport  Port=5
  Trajectory_capture : Outport  Port=6
  in_steep : Outport  Port=7
  In_round : Outport  Port=8
  Slight decline : Outport  Port=9
  in_flare : Outport  Port=10
  touch_ground : Outport  Port=11
  in_ground : Outport  Port=12
  h_ALG : Outport  Port=13
  e_psi : Outport  Port=14
  e_Y : Outport  Port=15
  stop_condition : Outport  Port=16
  wires:
  Compare To Constant8/1 -> Logical Operator2/2
  Compare To Constant7/1 -> Logical Operator2/1
  持续1秒/1(out) -> safe_climb/1
  Logical Operator2/1 -> 持续1秒/1(判断条件)  "安全爬升"
  Subsystem1/1(out) -> reach_VR/1
  Compare To Constant6/1 -> Subsystem1/1(判断条件)  "达到抬轮速度"
  Compare To Constant15/1 -> AND/1
  AND/1 -> Slight decline/1
  Compare To Constant17/1 -> AND/2
  AND1/1 -> In_round/1
  Compare To Constant14/1 -> AND1/1
  Compare To Constant18/1 -> AND1/2
  Compare To Constant16/1 -> AND2/1
  AND2/1 -> in_flare/1
  Compare To Constant19/1 -> AND2/2
  X/1 -> Compare To Constant2/1
  Compare To Constant20/1 -> in_steep/1
  [contact_right] -> AND4/2
  [contact_left] -> AND4/1
  AND3/1 -> in_ground/1  "进入13滑跑减速段"
  AND4/1 -> AND3/1, touch_ground/1  "进入12接地段"
  [no_contact] -> airborne/1  "进入爬升段"
  [vxg] -> Compare To Constant6/1
  [vzg] -> Gain1/1
  Gain/1 -> h_ALG/1, Compare To Constant7/1, Compare To Constant1/1, Compare To Constant19/1, Compare To Constant16/1, Compare To Constant17/1, Compare To Constant15/1, Compare To Constant18/1, Compare To Constant14/1, Compare To Constant20/1
  Compare To Constant1/1 -> 持续1秒1/1(判断条件)
  持续1秒1/1(out) -> in_cruise/1
  Z/1 -> Gain/1
  [contact_nose] -> AND3/2
  单位是弧度/1 -> AND5/2
  psi/1 -> e_psi/1, Abs1/1  "航航角偏差"
  Y/1 -> e_Y/1, Abs/1  "横向距离偏差"
  Abs/1 -> Compare To Constant9/1
  AND5/1 -> Trajectory_capture/1  "航向道截获"
  Abs1/1 -> 单位是弧度/1
  Compare To Constant9/1 -> AND5/1
  Compare To Constant2/1 -> Switch/2
  Switch/1 -> Scope/1, task_mode/1
  Constant/1 -> Switch/1
  Constant1/1 -> Switch/3
  Gain1/1 -> Compare To Constant8/1
  [Vg] -> Compare To Constant13/1
  Compare To Constant13/1 -> Subsystem2/1(判断条件)  "停稳"
  Subsystem2/1(out) -> stop_condition/1

== system A320_23b/Guidance/起飞阶段 ==
  Flight_phase : Inport
  e_Y : Inport  Port=2
  e_psi : Inport  Port=3
  r : Inport  Port=4
  Vwind_ground : Inport  Port=5
  Va_safe : Inport  Port=6
  h_ALG : Inport  Port=7
  vzg : Inport  Port=8
  phi_eular : Inport  Port=9
  theta_eular : Inport  Port=10
  Enable : EnablePort
  AND : Logic  IconShape=distinctive  AllPortsSameDT=off  OutDataTypeStr=boolean
  Compare To Constant : simulink/Logic and Bit Operations/Compare To Constant  relop===  const=1  OutDataTypeStr=boolean
  Compare To Constant1 : simulink/Logic and Bit Operations/Compare To Constant  relop=>=  const=2  OutDataTypeStr=boolean
  Compare To Constant2 : simulink/Logic and Bit Operations/Compare To Constant  relop=<=  const=4  OutDataTypeStr=boolean
  Compare To Constant3 : simulink/Logic and Bit Operations/Compare To Constant  relop===  const=5  OutDataTypeStr=boolean
  Merge : Merge  Inputs=3
  地面滑跑阶段(1) : Subsystem
  巡航阶段(5) : Subsystem  TreatAsAtomicUnit=on
  抬轮离地爬升阶段(2/3/4) : Subsystem  TreatAsAtomicUnit=on
  Cmd_Bus : Outport
  wires:
  抬轮离地爬升阶段(2/3/4)/1(Cmd_Bus) -> Merge/2
  地面滑跑阶段(1)/1(Cmd_Bus) -> Merge/1
  Merge/1 -> Cmd_Bus/1
  巡航阶段(5)/1(Cmd_Bus) -> Merge/3
  Flight_phase/1 -> Compare To Constant3/1, Compare To Constant2/1, Compare To Constant1/1, Compare To Constant/1
  Compare To Constant/1 -> 地面滑跑阶段(1)/Enable
  Compare To Constant1/1 -> AND/1
  Compare To Constant2/1 -> AND/2
  AND/1 -> 抬轮离地爬升阶段(2/3/4)/Enable
  Compare To Constant3/1 -> 巡航阶段(5)/Enable
  e_Y/1 -> 地面滑跑阶段(1)/1(e_Y)
  e_psi/1 -> 地面滑跑阶段(1)/2(e_psi)
  r/1 -> 地面滑跑阶段(1)/3(r)
  Vwind_ground/1 -> 抬轮离地爬升阶段(2/3/4)/1(Vwind_ground), 巡航阶段(5)/1(Vwind_ground)
  Va_safe/1 -> 巡航阶段(5)/2(Va_safe), 抬轮离地爬升阶段(2/3/4)/2(Va_safe)
  h_ALG/1 -> 巡航阶段(5)/3(h_ALG)
  vzg/1 -> 巡航阶段(5)/4(vzg)
  phi_eular/1 -> 巡航阶段(5)/5(phi_eular)
  theta_eular/1 -> 巡航阶段(5)/6(theta_eular)

== system A320_23b/Guidance/降落阶段 ==
  Flight_phase : Inport
  h_AGL : Inport  Port=2
  Vwind_ground : Inport  Port=3
  Va_safe : Inport  Port=4
  x_pos : Inport  Port=5
  vzg : Inport  Port=6
  phi_eular : Inport  Port=7
  theta_eular : Inport  Port=8
  Vg : Inport  Port=9
  Enable : EnablePort
  AND : Logic  IconShape=distinctive  AllPortsSameDT=off  OutDataTypeStr=boolean
  Compare To Constant : simulink/Logic and Bit Operations/Compare To Constant  relop=<=  const=7  OutDataTypeStr=boolean
  Compare To Constant1 : simulink/Logic and Bit Operations/Compare To Constant  relop=<=  const=10  OutDataTypeStr=boolean
  Compare To Constant2 : simulink/Logic and Bit Operations/Compare To Constant  relop=>  const=7  OutDataTypeStr=boolean
  Compare To Constant3 : simulink/Logic and Bit Operations/Compare To Constant  relop=>  const=10  OutDataTypeStr=boolean
  MATLAB Function : MATLAB Function  TreatAsAtomicUnit=on
  Merge : Merge  Inputs=3
  拉平/接地/滑跑刹车阶段(11/12/13) : Subsystem  TreatAsAtomicUnit=on
  进场/轨迹捕获阶段(6/7) : Subsystem  TreatAsAtomicUnit=on
  陡下滑/圆拉平/浅下滑阶段(8/9/10) : Subsystem  TreatAsAtomicUnit=on
  Cmd_Bus : Outport
  wires:
  陡下滑/圆拉平/浅下滑阶段(8/9/10)/1(Cmd_Bus) -> Merge/2
  x_pos/1 -> MATLAB Function/2(X)
  MATLAB Function/2(H_cmd) -> 进场/轨迹捕获阶段(6/7)/8(H_cmd), 陡下滑/圆拉平/浅下滑阶段(8/9/10)/9(H_cmd), 拉平/接地/滑跑刹车阶段(11/12/13)/3(H_cmd)
  Flight_phase/1 -> Compare To Constant1/1, Compare To Constant2/1, 拉平/接地/滑跑刹车阶段(11/12/13)/1(Flight_Phase), Compare To Constant3/1, 陡下滑/圆拉平/浅下滑阶段(8/9/10)/3(Flight_phase), Compare To Constant/1, MATLAB Function/1(Flight_Phase)
  Merge/1 -> Cmd_Bus/1
  Compare To Constant2/1 -> AND/2
  vzg/1 -> 进场/轨迹捕获阶段(6/7)/4(vzg), 陡下滑/圆拉平/浅下滑阶段(8/9/10)/5(vzg)
  AND/1 -> 陡下滑/圆拉平/浅下滑阶段(8/9/10)/Enable
  h_AGL/1 -> 进场/轨迹捕获阶段(6/7)/3(h_ALG), 陡下滑/圆拉平/浅下滑阶段(8/9/10)/4(h_ALG), MATLAB Function/3(h_AGL)
  theta_eular/1 -> 陡下滑/圆拉平/浅下滑阶段(8/9/10)/7(theta_eular), 进场/轨迹捕获阶段(6/7)/6(theta_eular)
  Vwind_ground/1 -> 进场/轨迹捕获阶段(6/7)/1(Vwind_ground), 陡下滑/圆拉平/浅下滑阶段(8/9/10)/1(Vwind_ground), 拉平/接地/滑跑刹车阶段(11/12/13)/4(Vwind_ground)
  MATLAB Function/1(gamma_cmd) -> 拉平/接地/滑跑刹车阶段(11/12/13)/2(gamma_cmd), 陡下滑/圆拉平/浅下滑阶段(8/9/10)/8(gamma_cmd), 进场/轨迹捕获阶段(6/7)/7(gamma_cmd)
  phi_eular/1 -> 陡下滑/圆拉平/浅下滑阶段(8/9/10)/6(phi_eular), 进场/轨迹捕获阶段(6/7)/5(phi_eular)
  Vg/1 -> MATLAB Function/4(Vg)
  进场/轨迹捕获阶段(6/7)/1(Cmd_Bus) -> Merge/1
  Compare To Constant1/1 -> AND/1
  拉平/接地/滑跑刹车阶段(11/12/13)/1(Cmd_Bus) -> Merge/3
  Compare To Constant/1 -> 进场/轨迹捕获阶段(6/7)/Enable
  Compare To Constant3/1 -> 拉平/接地/滑跑刹车阶段(11/12/13)/Enable
  Va_safe/1 -> 进场/轨迹捕获阶段(6/7)/2(Va_safe), 拉平/接地/滑跑刹车阶段(11/12/13)/5(Va_safe), 陡下滑/圆拉平/浅下滑阶段(8/9/10)/2(Va_safe)

== system A320_23b/controller1/1_Pitch_Ctrl ==
  Flight_Phase : Inport
  nz_cmd : Inport  Port=2
  theta_cmd : Inport  Port=3
  nz : Inport  Port=4
  theta : Inport  Port=5
  q : Inport  Port=6
  H_cmd : Inport  Port=7
  gamma : Inport  Port=8
  234俯仰角控制 : Subsystem
  567C*控制 : Subsystem
  89101112_着陆俯仰控制 : Subsystem
  Clock_blend : Clock
  Compare To Constant : simulink/Logic and Bit Operations/Compare To Constant  relop=>=  const=2  OutDataTypeStr=boolean
  Compare To Constant1 : simulink/Logic and Bit Operations/Compare To Constant  relop===  const=6  OutDataTypeStr=boolean
  Compare To Constant2 : simulink/Logic and Bit Operations/Compare To Constant  relop=<=  const=5  OutDataTypeStr=boolean
  Compare To Constant3 : simulink/Logic and Bit Operations/Compare To Constant  relop=>=  const=8  OutDataTypeStr=boolean
  Compare To Constant4 : simulink/Logic and Bit Operations/Compare To Constant  relop===  const=7  OutDataTypeStr=boolean
  Compare To Constant5 : simulink/Logic and Bit Operations/Compare To Constant  relop===  const=5  OutDataTypeStr=boolean
  Compare To Constant6 : simulink/Logic and Bit Operations/Compare To Constant  relop===  const=6  OutDataTypeStr=boolean
  Compare To Constant7 : simulink/Logic and Bit Operations/Compare To Constant  relop===  const=7  OutDataTypeStr=boolean
  Compare To Constant8 : simulink/Logic and Bit Operations/Compare To Constant  relop=<=  const=12  OutDataTypeStr=boolean
  Constant : Constant  Value=0
  Gain3 : Gain  Gain=HD
  Gain4 : Gain  Gain=HD
  Logical Operator : Logic  AllPortsSameDT=off  OutDataTypeStr=boolean
  Logical Operator1 : Logic  AllPortsSameDT=off  OutDataTypeStr=boolean
  Logical Operator2 : Logic  Operator=NOT  AllPortsSameDT=off  OutDataTypeStr=boolean
  Logical Operator3 : Logic  Operator=OR  AllPortsSameDT=off  OutDataTypeStr=boolean
  Logical Operator4 : Logic  Operator=OR  Inputs=3  AllPortsSameDT=off  OutDataTypeStr=boolean
  Pitch45Blend : MATLAB Function  TreatAsAtomicUnit=on  SystemSampleTime=0.001
  Saturation : Saturate  UpperLimit=25  LowerLimit=-25
  Scope1 : Scope
  Switch : Switch  Criteria=u2 > Threshold  SaturateOnIntegerOverflow=off  InputSameDT=off
  Switch1 : Switch  Criteria=u2 > Threshold  SaturateOnIntegerOverflow=off  InputSameDT=off
  Switch2 : Switch  Criteria=u2 > Threshold  SaturateOnIntegerOverflow=off  InputSameDT=off
  T_blend : Constant  Value=5
  de_cmd : Outport
  wires:
  Flight_Phase/1 -> Compare To Constant5/1, Compare To Constant1/1, Compare To Constant8/1, Compare To Constant3/1, Compare To Constant4/1, Compare To Constant6/1, Compare To Constant7/1, Pitch45Blend/1(phase), Compare To Constant/1, Compare To Constant2/1
  Gain3/1 -> Saturation/1
  theta_cmd/1 -> 234俯仰角控制/1(theta_cmd)
  theta/1 -> 234俯仰角控制/2(theta)
  nz_cmd/1 -> 567C*控制/1(nz_cmd)
  nz/1 -> 567C*控制/2(nz)
  q/1 -> 234俯仰角控制/3(q), 567C*控制/3(q)
  567C*控制/1(de_nz_rad) -> Gain4/1, Pitch45Blend/3(de_ny_rad)
  Compare To Constant1/1 -> Logical Operator3/2
  Compare To Constant4/1 -> Logical Operator3/1
  Logical Operator3/1 -> Switch/2
  [Vg] -> 89101112_着陆俯仰控制/1(Vg)
  H_cmd/1 -> 89101112_着陆俯仰控制/3(h_cmd)
  gamma/1 -> 89101112_着陆俯仰控制/2(gamma)
  Compare To Constant6/1 -> Logical Operator4/2
  Compare To Constant7/1 -> Logical Operator4/1
  Logical Operator4/1 -> Logical Operator2/1
  Compare To Constant5/1 -> Logical Operator4/3
  Gain4/1 -> Switch/1
  Compare To Constant/1 -> Logical Operator/1
  Compare To Constant2/1 -> Logical Operator/2
  Logical Operator/1 -> Switch1/2
  234俯仰角控制/1(de_theta_rad) -> Pitch45Blend/2(de_theta_rad)
  Clock_blend/1 -> Pitch45Blend/4(t)
  T_blend/1 -> Pitch45Blend/5(T_blend)
  Pitch45Blend/1(de_cmd_rad) -> Gain3/1
  Saturation/1 -> Switch1/1
  Pitch45Blend/2(lambda) -> Scope1/1
  Switch/1 -> Switch1/3
  Switch1/1 -> de_cmd/1
  Switch2/1 -> Switch/3
  Logical Operator1/1 -> Switch2/2
  Compare To Constant3/1 -> Logical Operator1/1
  Compare To Constant8/1 -> Logical Operator1/2
  89101112_着陆俯仰控制/1(de(D)) -> Switch2/1
  Constant/1 -> Switch2/3

== system A320_23b/controller1/2_Yaw_Ctrl ==
  Flight_Phase : Inport
  Y : Inport  Port=2
  psi : Inport  Port=3
  r : Inport  Port=4
  psi_cmd : Inport  Port=5
  23456789101112段控制 : Subsystem
  Compare To Constant : simulink/Logic and Bit Operations/Compare To Constant  relop=>=  const=2  OutDataTypeStr=boolean
  Compare To Constant1 : simulink/Logic and Bit Operations/Compare To Constant  relop=<=  const=12  OutDataTypeStr=boolean
  Compare To Constant2 : simulink/Logic and Bit Operations/Compare To Constant  relop===  const=1  OutDataTypeStr=boolean
  Compare To Constant4 : simulink/Logic and Bit Operations/Compare To Constant  relop===  const=13  OutDataTypeStr=boolean
  Constant : Constant  Value=0
  Constant1 : Constant  Value=0
  Constant2 : Constant  Value=0
  Gain : Gain  Gain=HD
  Gain1 : Gain  Gain=HD
  Gain2 : Gain  Gain=-0.2
  Gain3 : Gain  Gain=-0.85
  K_z : Constant  Value=0.08
  Logical Operator : Logic  AllPortsSameDT=off  OutDataTypeStr=boolean
  Logical Operator1 : Logic  Operator=OR  AllPortsSameDT=off  OutDataTypeStr=boolean
  Product : Product
  Saturation : Saturate  UpperLimit=25  LowerLimit=-25
  Saturation1 : Saturate  UpperLimit=25  LowerLimit=-25
  Scope1 : Scope
  Sum : Sum  Inputs=|+-
  Sum1 : Sum  Inputs=|++
  Sum3 : Sum  Inputs=|++
  Switch : Switch  Criteria=u2 > Threshold  SaturateOnIntegerOverflow=off  InputSameDT=off
  Switch1 : Switch  Criteria=u2 > Threshold  SaturateOnIntegerOverflow=off  InputSameDT=off
  dr_cmd : Outport
  delta_s_cmd : Outport  Port=2
  wires:
  Gain/1 -> Saturation/1
  Saturation/1 -> dr_cmd/1
  Saturation1/1 -> delta_s_cmd/1
  Gain1/1 -> Saturation1/1
  Compare To Constant/1 -> Logical Operator/1
  Compare To Constant1/1 -> Logical Operator/2
  Logical Operator/1 -> Switch/2
  Compare To Constant2/1 -> Logical Operator1/1
  Logical Operator1/1 -> Switch1/2
  Constant/1 -> Switch1/3
  Flight_Phase/1 -> Compare To Constant/1, Compare To Constant1/1, Compare To Constant2/1, Compare To Constant4/1
  Constant1/1 -> Switch/3
  Switch1/1 -> Gain1/1
  Switch/1 -> Gain/1
  23456789101112段控制/1(dr_cmd) -> Switch/1
  Y/1 -> Sum/2, Scope1/1, 23456789101112段控制/1(Y)
  psi/1 -> Gain3/1, 23456789101112段控制/2(psi)
  r/1 -> Gain2/1, 23456789101112段控制/3(r)
  Gain3/1 -> Sum1/2
  Sum1/1 -> Sum3/1
  Gain2/1 -> Sum3/2
  Constant2/1 -> Sum/1
  Product/1 -> Sum1/1
  Sum/1 -> Product/2
  K_z/1 -> Product/1
  Sum3/1 -> Switch1/1
  Compare To Constant4/1 -> Logical Operator1/2
  psi_cmd/1 -> 23456789101112段控制/4(psi_cmd)

== system A320_23b/controller1/3_Roll_Ctrl ==
  phi_cmd : Inport
  phi : Inport  Port=2
  p : Inport  Port=3
  Gain : Gain  Gain=180/pi
  Gain1 : Gain
  Gain2 : Gain  Gain=5
  Gain3 : Gain  Gain=0.1
  Gain4 : Gain  Gain=-1
  Integrator : Integrator
  Saturation : Saturate  UpperLimit=25  LowerLimit=-25
  Saturation1 : Saturate  UpperLimit=0.52  LowerLimit=-0.52
  Sum : Sum  Inputs=|+-
  Sum1 : Sum  Inputs=|++
  Sum2 : Sum  Inputs=|+-
  da_cmd : Outport
  wires:
  Gain/1 -> Saturation/1
  Saturation/1 -> Gain4/1
  phi_cmd/1 -> Sum/1
  phi/1 -> Sum/2
  Sum/1 -> Saturation1/1
  Gain3/1 -> Integrator/1
  Integrator/1 -> Sum1/2
  Gain2/1 -> Sum1/1
  Sum1/1 -> Sum2/1
  p/1 -> Sum2/2
  Sum2/1 -> Gain1/1
  Saturation1/1 -> Gain2/1, Gain3/1
  Gain1/1 -> Gain/1
  Gain4/1 -> da_cmd/1

== system A320_23b/controller1/4_Power&V_Ctrl ==
  Flight_Phase : Inport
  throttle_cmd : Inport  Port=2
  V_cmd : Inport  Port=3
  V : Inport  Port=4
  brake_cmd : Inport  Port=5
  Clock_blend : Clock
  Compare To Constant1 : simulink/Logic and Bit Operations/Compare To Constant  relop=>=  const=1  OutDataTypeStr=boolean
  Compare To Constant2 : simulink/Logic and Bit Operations/Compare To Constant  relop=<=  const=5  OutDataTypeStr=boolean
  Compare To Constant3 : simulink/Logic and Bit Operations/Compare To Constant  relop=>=  const=6  OutDataTypeStr=boolean
  Compare To Constant5 : simulink/Logic and Bit Operations/Compare To Constant  relop=<=  const=12  OutDataTypeStr=boolean
  Constant : Constant  Value=5
  Constant3 : Constant  Value=0
  Delay1 : Delay  DelayLength=1
  Gain2 : Gain  Gain=0.1
  Gain3 : Gain  Gain=0.08
  Logical Operator : Logic  AllPortsSameDT=off  OutDataTypeStr=boolean
  Logical Operator1 : Logic  AllPortsSameDT=off  OutDataTypeStr=boolean
  MATLAB Function1 : MATLAB Function  TreatAsAtomicUnit=on
  MATLAB Function2 : MATLAB Function  TreatAsAtomicUnit=on
  Saturation1 : Saturate  UpperLimit=1  LowerLimit=0
  Saturation2 : Saturate  UpperLimit=1  LowerLimit=0
  Saturation3 : Saturate  UpperLimit=0.55  LowerLimit=-0.45
  Scope : Scope
  Sum4 : Sum  Inputs=|+-
  Sum5 : Sum  Inputs=|++
  Sum6 : Sum  Inputs=|+-
  Switch1 : Switch  Criteria=u2 > Threshold  SaturateOnIntegerOverflow=off  InputSameDT=off
  Switch2 : Switch  Criteria=u2 > Threshold  SaturateOnIntegerOverflow=off  InputSameDT=off
  平衡油门 : Constant  Value=0.3
  throttle : Outport
  u_brake_cmd : Outport  Port=2
  wires:
  Saturation1/1 -> u_brake_cmd/1
  brake_cmd/1 -> Saturation1/1
  Compare To Constant1/1 -> Logical Operator/1
  Compare To Constant2/1 -> Logical Operator/2
  Flight_Phase/1 -> MATLAB Function1/1(phase), Compare To Constant3/1, Compare To Constant5/1, Compare To Constant2/1, Compare To Constant1/1
  平衡油门/1 -> Sum5/2
  V/1 -> Sum6/2
  Sum6/1 -> Gain2/1
  Gain2/1 -> Sum4/1
  V_cmd/1 -> Sum6/1
  Sum4/1 -> Saturation3/1
  [vg_xyz] -> MATLAB Function2/1(Vel_g)
  Saturation3/1 -> Sum5/1
  Delay1/1 -> Gain3/1
  Sum5/1 -> MATLAB Function1/3(throttle_speed), Switch1/1
  MATLAB Function2/1(dv_err) -> Delay1/1
  Gain3/1 -> Sum4/2
  [a_xyz] -> MATLAB Function2/2(axyz)
  MATLAB Function1/1(throttle_out) -> Saturation2/1
  Clock_blend/1 -> MATLAB Function1/4(t)
  Constant/1 -> MATLAB Function1/5(T_blend)
  throttle_cmd/1 -> MATLAB Function1/2(throttle_direct)
  MATLAB Function1/2(lambda) -> Scope/1
  Logical Operator/1 -> Switch2/2
  Saturation2/1 -> Switch2/1
  Switch1/1 -> Switch2/3
  Logical Operator1/1 -> Switch1/2
  Compare To Constant3/1 -> Logical Operator1/1
  Compare To Constant5/1 -> Logical Operator1/2
  Constant3/1 -> Switch1/3
  Switch2/1 -> throttle/1

== system A320_23b/controller1/刹车 ==
  u_brake_cmd : Inport
  Gain : Gain  Gain=1/0.1
  Integrator : Integrator  LimitOutput=on  UpperSaturationLimit=1  LowerSaturationLimit=0
  Sum : Sum  Inputs=|+-
  限制舵面角速度 : Saturate  UpperLimit=5  LowerLimit=-5
  u_brake : Outport
  wires:
  u_brake_cmd/1 -> Sum/1
  Sum/1 -> Gain/1
  Gain/1 -> 限制舵面角速度/1
  限制舵面角速度/1 -> Integrator/1
  Integrator/1 -> Sum/2, u_brake/1

== system A320_23b/controller1/前轮 ==
  delta_s_cmd : Inport
  Gain : Gain  Gain=1/0.08
  Integrator : Integrator  LimitOutput=on  UpperSaturationLimit=25  LowerSaturationLimit=-25
  Sum : Sum  Inputs=|+-
  限制偏转速度 : Saturate  UpperLimit=120  LowerLimit=-120
  delta_s : Outport
  wires:
  delta_s_cmd/1 -> Sum/1
  Sum/1 -> Gain/1
  Gain/1 -> 限制偏转速度/1
  限制偏转速度/1 -> Integrator/1
  Integrator/1 -> Sum/2, delta_s/1

== system A320_23b/controller1/副翼 ==
  da_cmd : Inport
  Gain : Gain  Gain=1/0.05
  Integrator : Integrator  LimitOutput=on  UpperSaturationLimit=25  LowerSaturationLimit=-25
  Sum : Sum  Inputs=|+-
  限制舵面角速度 : Saturate  UpperLimit=120  LowerLimit=-120
  da : Outport
  wires:
  da_cmd/1 -> Sum/1
  Sum/1 -> Gain/1
  Gain/1 -> 限制舵面角速度/1
  限制舵面角速度/1 -> Integrator/1
  Integrator/1 -> Sum/2, da/1

== system A320_23b/controller1/升降舵 ==
  de_cmd : Inport
  Gain : Gain  Gain=1/0.08
  Integrator : Integrator  LimitOutput=on  UpperSaturationLimit=25  LowerSaturationLimit=-25
  Sum : Sum  Inputs=|+-
  限制舵面角速度 : Saturate  UpperLimit=50  LowerLimit=-50
  de : Outport
  wires:
  de_cmd/1 -> Sum/1
  Sum/1 -> Gain/1
  Gain/1 -> 限制舵面角速度/1
  限制舵面角速度/1 -> Integrator/1
  Integrator/1 -> Sum/2, de/1

== system A320_23b/controller1/方向舵 ==
  dr_cmd : Inport
  Gain : Gain  Gain=1/0.05
  Integrator : Integrator  LimitOutput=on  UpperSaturationLimit=25  LowerSaturationLimit=-25
  Sum : Sum  Inputs=|+-
  限制舵面角速度 : Saturate  UpperLimit=100  LowerLimit=-100
  dr : Outport
  wires:
  Integrator/1 -> dr/1, Sum/2
  限制舵面角速度/1 -> Integrator/1
  Gain/1 -> 限制舵面角速度/1
  Sum/1 -> Gain/1
  dr_cmd/1 -> Sum/1

== system A320_23b/controller1/油门 ==
  throttle : Inport
  Gain : Gain  Gain=1/0.5
  Integrator : Integrator  LimitOutput=on  UpperSaturationLimit=1  LowerSaturationLimit=0
  Saturation : Saturate  UpperLimit=3  LowerLimit=-3
  Sum : Sum  Inputs=|+-
  up : Outport
  wires:
  Saturation/1 -> Integrator/1
  Gain/1 -> Saturation/1
  Sum/1 -> Gain/1
  throttle/1 -> Sum/1
  Integrator/1 -> up/1, Sum/2

== system A320_23b/6DOF-MODEL/AERO-PARAMETER/atmosphere ==
  Add : Sum
  Band-Limited White Noise : simulink/Sources/Band-Limited White Noise  Cov=[1]  Ts=0.1  seed=[23341]
  Constant1 : Constant  Value=rho0
  Constant2 : Constant  Value=a0
  Constant3 : Constant  Value=0.5
  Constant4 : Constant  Value=0
  Constant5 : Constant  Value=0
  Constant6 : Constant  Value=5
  Display : Display
  Gain : Gain
  MATLAB Function : MATLAB Function  TreatAsAtomicUnit=on
  Matrix Multiply : Product  Multiplication=Matrix(*)
  Mux : Mux  Inputs=3
  Product : Product  Inputs=3
  Reshape : Reshape  OutputDimensionality=Column vector (2-D)
  Scope : Scope
  Square : Math  Operator=square
  Transfer Fcn : TransferFcn  Denominator=[10 1]
  tag scope: Vwind_body=global, Vwind_ground=global, a_sound=global, qc=global, rho=global
  wires:
  Constant1/1 -> [rho]
  Constant2/1 -> [a_sound]
  Constant3/1 -> Product/1
  [rho] -> Product/2
  Product/1 -> Display/1, [qc]
  Square/1 -> Product/3
  [Vg] -> Square/1
  Reshape/1 -> [Vwind_ground]
  [Vwind_ground] -> Matrix Multiply/2
  [theta_eular] -> MATLAB Function/2(theta)
  [phi_eular] -> MATLAB Function/1(phi)
  MATLAB Function/1(R_bg) -> Matrix Multiply/1
  [psi_eular] -> MATLAB Function/3(psi)
  Matrix Multiply/1 -> [Vwind_body]
  Gain/1 -> Add/1
  Transfer Fcn/1 -> Gain/1
  Band-Limited White Noise/1 -> Transfer Fcn/1
  Constant5/1 -> Mux/3
  Constant4/1 -> Mux/1
  Add/1 -> Scope/1, Mux/2
  Constant6/1 -> Add/2

== system A320_23b/6DOF-MODEL/AERO-PARAMETER/侧向力系数 ==
  beta(H) : Inport
  dr(H) : Inport  Port=2
  Add : Sum  Inputs=++++
  CYpConst : Constant  Value=CYp
  CYpXPhat : Product
  Constant1 : Constant  Value=CSb
  Constant2 : Constant  Value=CSr
  Constant3 : Constant  Value=CSdr
  Product : Product
  Product2 : Product
  Product3 : Product
  CS : Outport
  wires:
  Add/1 -> CS/1
  Constant3/1 -> Product2/2
  Product2/1 -> Add/3
  dr(H)/1 -> Product2/1
  beta(H)/1 -> Product/1
  Constant1/1 -> Product/2
  Constant2/1 -> Product3/2
  [r_hat] -> Product3/1
  Product/1 -> Add/1
  Product3/1 -> Add/2
  [p_hat] -> CYpXPhat/1
  CYpConst/1 -> CYpXPhat/2
  CYpXPhat/1 -> Add/4
